simulink model "model_2dof_test"  (R2024b)
settings: Solver=VariableStepAuto  StartTime=0.0  StopTime=10.0  RelTol=1e-3
values from neighbouring files (symbols this model uses):
  Ct = 2.0e8    (= 200000000)    [check_2dof_model.m]    (also in ex9.m = 210000000; load_ex9_model.m)
  Dr = 0    [check_2dof_model.m]    (also in ex8_4.m; ex9.m; load_ex9_model.m)
  Jr = 3.0e-2    (= 0.03)    [check_2dof_model.m]    (also in ex9.m; load_ex9_model.m; load_params.m = 0.00222)
  KT = 1    [check_2dof_model.m]    (also in ex8_4.m; ex9.m; load_ex9_model.m)
  Kt = 1.0e8    (= 100000000)    [check_2dof_model.m]    (also in ex9.m; load_ex9_model.m; load_params.m = 110000000)
  Mt = 100    [check_2dof_model.m]    (also in ex9.m = 200; load_ex9_model.m; load_params.m = 500)
  R = lp/2/pi    (= 0.00159154943092)    [check_2dof_model.m]    (also in ex9.m; load_ex9_model.m; load_params.m = 0.0032)
settings Model: Creator=shohei  LastModifiedBy=shohei

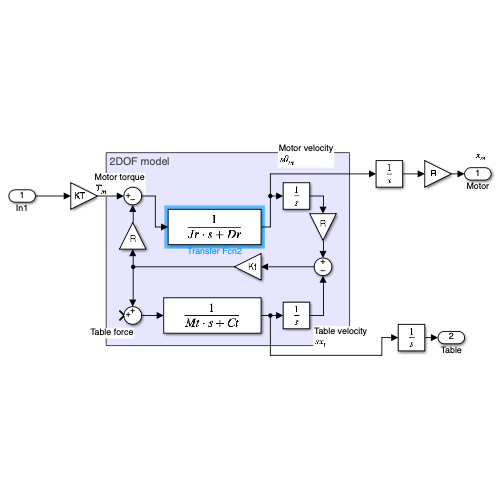
[thumbnail: Simulink's stored preview of the top-level diagram]
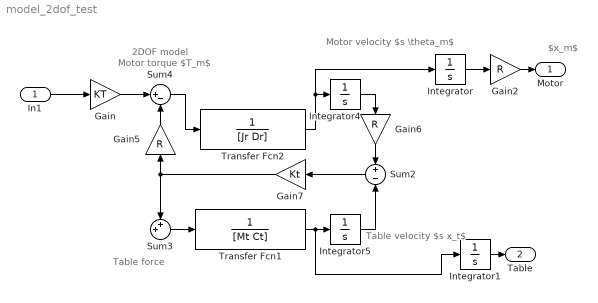
== system model_2dof_test ==
  note: Motor velocity
      | $s \theta_m$
  note: Table velocity
      | $s x_t$
  note: 2DOF model
  note: Motor torque
      | $T_m$
  note: Table force
  note: $x_m$
  In1 : Inport
  Gain : Gain  Gain=KT
  Gain2 : Gain  Gain=R
  Gain5 : Gain  Gain=R
  Gain6 : Gain  Gain=R
  Gain7 : Gain  Gain=Kt
  Integrator{,1,4..5} (4 alike) : Integrator
  Sum2 : Sum  Inputs=+|-
  Sum3 : Sum  Inputs=++|
  Sum4 : Sum  Inputs=|+-
  Transfer Fcn1 : TransferFcn  Denominator=[Mt Ct]
  Transfer Fcn2 : TransferFcn  Denominator=[Jr Dr]
  Motor : Outport
  Table : Outport  Port=2
  wires:
  Gain6/1 -> Sum2/1
  Sum2/1 -> Gain7/1
  Transfer Fcn1/1 -> Integrator1/1, Integrator5/1
  Transfer Fcn2/1 -> Integrator/1, Integrator4/1
  Gain7/1 -> Sum3/1, Gain5/1
  Sum4/1 -> Transfer Fcn2/1
  Gain5/1 -> Sum4/2
  Integrator5/1 -> Sum2/2
  Gain/1 -> Sum4/1
  Integrator4/1 -> Gain6/1
  Sum3/1 -> Transfer Fcn1/1
  Gain2/1 -> Motor/1
  Integrator/1 -> Gain2/1
  Integrator1/1 -> Table/1
  In1/1 -> Gain/1
